simulink model "PwmGenerator"  (R2025a)
settings: Solver=VariableStepAuto  StartTime=0.0  StopTime=10.0  RelTol=1e-3
undefined symbols (not defined in the file): TTL_amplitude
settings Model: DataDictionary=PwmGenerator.sldd  Creator=tecnicomcbti  LastModifiedBy=tecnicomcbti

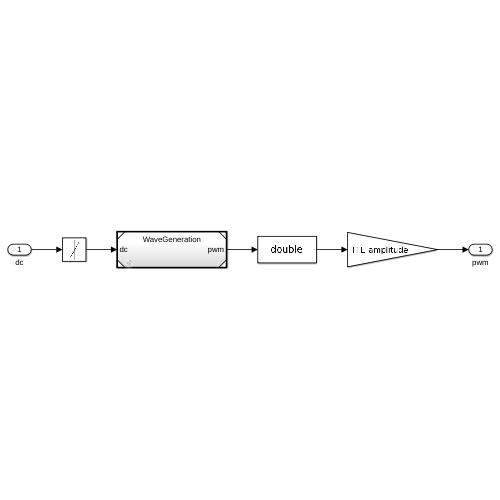
[thumbnail: Simulink's stored preview of the top-level diagram]
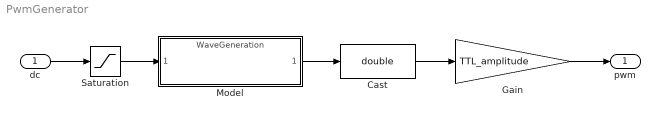
== system PwmGenerator ==
  dc : Inport
  Cast : DataTypeConversion  OutDataTypeStr=double  SaturateOnIntegerOverflow=off  RndMeth=Floor
  Gain : Gain  Gain=TTL_amplitude
  Model : ModelReference  ModelNameDialog=WaveGeneration.slx  SimulationMode=Normal  ModelReferenceVersion=1.5
  Saturation : Saturate  UpperLimit=1  LowerLimit=0
  pwm : Outport
  wires:
  Cast/1 -> Gain/1
  dc/1 -> Saturation/1
  Gain/1 -> pwm/1
  Saturation/1 -> Model/1
  Model/1 -> Cast/1
